simulink model "Lazurit_zarud_V2"  (R2018b)
settings: Solver=VariableStepAuto  StartTime=0.0  StopTime=2.5  RelTol=1e-3
undefined symbols (not defined in the file): Cout_filter_c, Cout_filter_r, Czpt_c, Czpt_r, delay_module_2, DiscIntNeverNeededParam, f, L_l, L_r, Lzpt_l, Lzpt_r, Rout, Ul, Uout, Uzpt
libraries: powerlib x60, powerlib_meascontrol x16, dspstat3 x11, simulink x4, simulink_extras x4, peRmsMeasurement x4
settings Model: Creator=VID Company  LastModifiedBy=VID Company

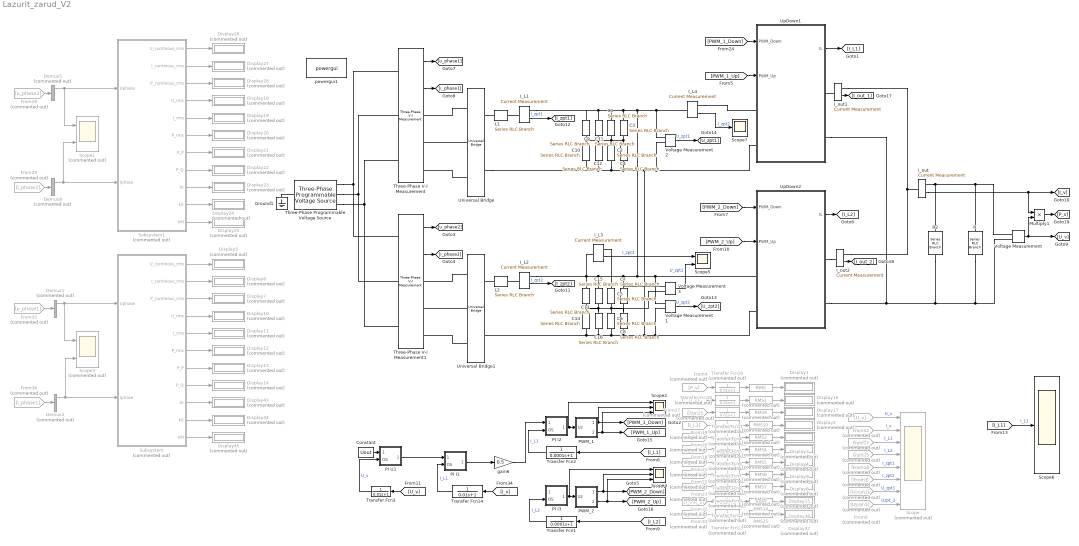
== system Lazurit_zarud_V2 ==
  C{1..16} (16 alike) : powerlib/Elements/Series RLC Branch  LConnTagsString=__new0  RConnTagsString=__new0  BranchType=RC  Resistance=Czpt_r  Inductance=1e-3  SetiL0=off  InitialCurrent=0  Capacitance=Czpt_c  Setx0=on  InitialVoltage=Uzpt/2  Measurements=Branch voltage
      settings: SourceProductName=Simscape Electrical
  Constant : Constant  Value=Uout
  Demux{1..2,5,8} (4 alike) : Demux  Commented=on  Outputs=3
  Display{1..28,37..38,43..45} (33 alike) : Display  Commented=on
  From1 : From  Commented=on  GotoTag=I_zpt1
  From12 : From  Commented=on  GotoTag=U_v
  From15 : From  Commented=on  GotoTag=I_L1
  From16 : From  Commented=on  GotoTag=I_L2
  From17 : From  Commented=on  GotoTag=I_v
  From18 : From  Commented=on  GotoTag=I_zpt1
  From19 : From  Commented=on  GotoTag=I_L1
  From2 : From  Commented=on  GotoTag=I_zpt2
  From20 : From  Commented=on  GotoTag=I_L2
  From21 : From  Commented=on  GotoTag=I_zpt2
  From22 : From  Commented=on  GotoTag=U_zpt1
  From23 : From  Commented=on  GotoTag=U_zpt2
  From25 : From  Commented=on  GotoTag=I_v
  From27 : From  Commented=on  GotoTag=U_v
  From28 : From  Commented=on  GotoTag=u_phase2
  From29 : From  Commented=on  GotoTag=i_phase2
  From3 : From  Commented=on  GotoTag=U_zpt1
  From32 : From  Commented=on  GotoTag=I_out_1
  From33 : From  Commented=on  GotoTag=I_out_2
  From35 : From  Commented=on  GotoTag=u_phase1
  From36 : From  Commented=on  GotoTag=i_phase1
  From4 : From  Commented=on  GotoTag=P_v
  From6 : From  Commented=on  GotoTag=U_zpt2
  Ground1 : powerlib/Elements/Ground  LConnTagsString=a
  I_L{1..4} (4 alike) : powerlib/Measurements/Current Measurement  PhasorSimulation=off  OutputType=Complex  PSBequivalent=0
      settings: SourceProductName=Simscape Electrical
  I_out : powerlib/Measurements/Current Measurement  PhasorSimulation=off  OutputType=Complex  PSBequivalent=0
      settings: SourceProductName=Simscape Electrical
  I_out1 : powerlib/Measurements/Current Measurement  PhasorSimulation=off  OutputType=Complex  PSBequivalent=0
      settings: SourceProductName=Simscape Electrical
  I_out2 : powerlib/Measurements/Current Measurement  PhasorSimulation=off  OutputType=Complex  PSBequivalent=0
      settings: SourceProductName=Simscape Electrical
  L1 : powerlib/Elements/Series RLC Branch  LConnTagsString=__new0  RConnTagsString=__new0  BranchType=RL  Resistance=Lzpt_r  Inductance=Lzpt_l  SetiL0=off  InitialCurrent=0  Capacitance=1e-6  Setx0=off  InitialVoltage=0  Measurements=None
      settings: SourceProductName=Simscape Electrical
  L2 : powerlib/Elements/Series RLC Branch  LConnTagsString=__new0  RConnTagsString=__new0  BranchType=RL  Resistance=Lzpt_r  Inductance=Lzpt_l  SetiL0=off  InitialCurrent=0  Capacitance=1e-6  Setx0=off  InitialVoltage=0  Measurements=None
      settings: SourceProductName=Simscape Electrical
  Multiply1 : Product
  PI I1 : Subsystem
  PI I2 : Subsystem
  PI I3 : Subsystem
  PI U1 : Subsystem
  PWM_1 : Subsystem
  PWM_2 : Subsystem
  R : powerlib/Elements/Series RLC Branch  LConnTagsString=__new0  RConnTagsString=__new0  BranchType=R  Resistance=Rout  Inductance=1e-3  SetiL0=off  InitialCurrent=0  Capacitance=6000e-6  Setx0=off  InitialVoltage=0  Measurements=None
  R2 : powerlib/Elements/Series RLC Branch  LConnTagsString=__new0  RConnTagsString=__new0  BranchType=R  Resistance=500  Inductance=1e-3  SetiL0=off  InitialCurrent=0  Capacitance=6000e-6  Setx0=off  InitialVoltage=0  Measurements=None
  RMS{1,3..10,14..15} (11 alike) : dspstat3/RMS  Commented=on  run=off  directionMode=Each column  dimension=1  InputProcessing=Columns as channels (frame based)  reset_popup=None
  Scope : Scope  Commented=on  NumInputPorts=8
  Scope1 : Scope  Commented=on  NumInputPorts=2
  Scope2 : Scope  NumInputPorts=3
  Scope3 : Scope  Commented=on  NumInputPorts=2
  Scope4 : Scope  NumInputPorts=3
  Scope5 : Scope  NumInputPorts=2
  Scope6 : Scope
  Scope7 : Scope
  Subsystem : Subsystem  Commented=on
  Subsystem1 : Subsystem  Commented=on
  Three-Phase Programmable Voltage Source : powerlib/Electrical Sources/Three-Phase Programmable Voltage Source  PositiveSequence=[Ul 0 50]  VariationEntity=None  VariationType=Table of time-amplitude pairs  VariationTypeAlt=Step  VariationStep=0.5  VariationRate=10  VariationMagnitude=0.3  VariationFrequency=2  VariationTiming=[1 2]  VariationPhaseA=off  Amplitudes=[1 0.8 1.2 1.0]  TimeValues=[0 0.1 0.15 0.2]  HarmonicGeneration=off  HarmonicA=[3 0.2 -25 0]  HarmonicB=[2 0.15 35 2]  Timing="[0.05  3]"  BusType=swing  Pref=0  Qref=0  Qmin=-inf  Qmax=inf
  Three-Phase V-I Measurement : powerlib/Measurements/Three-Phase V-I Measurement  VoltageMeasurement=phase-to-ground  SetLabelV=off  LabelV=Vabc  Vpu=off  VpuLL=off  CurrentMeasurement=yes  SetLabelI=off  LabelI=Iabc  Ipu=off  Pbase=100e6  Vbase=500e3  OutputType=Complex  PhasorSimulation=off  PSBequivalent=0
  Three-Phase V-I Measurement1 : powerlib/Measurements/Three-Phase V-I Measurement  VoltageMeasurement=phase-to-ground  SetLabelV=off  LabelV=Vabc  Vpu=off  VpuLL=off  CurrentMeasurement=yes  SetLabelI=off  LabelI=Iabc  Ipu=off  Pbase=100e6  Vbase=500e3  OutputType=Complex  PhasorSimulation=off  PSBequivalent=0
  Transfer Fcn1 : TransferFcn  Denominator=[0.0001 1]
  Transfer Fcn{4..13,19} (11 alike) : TransferFcn  Commented=on  Denominator=[0.01 1]
  Transfer Fcn14 : TransferFcn  Denominator=[0.01 1]
  Transfer Fcn2 : TransferFcn  Denominator=[0.0001 1]
  Transfer Fcn3 : TransferFcn  Denominator=[0.01 1]
  Universal Bridge : powerlib/Power Electronics/Universal Bridge  Arms=3  SnubberResistance=1e5  SnubberCapacitance=inf  Device=Diodes  Ron=Vd_r  Lon=0  ForwardVoltages="[  0  0  ]"  ForwardVoltage=Vd_v  GTOparameters=[ 10e-6 , 20e-6 ]  IGBTparameters=[ 1e-6 , 2e-6 ]  Measurements=None  Measurements_2=None  converterType=Rectifier
  Universal Bridge1 : powerlib/Power Electronics/Universal Bridge  Arms=3  SnubberResistance=1e5  SnubberCapacitance=inf  Device=Diodes  Ron=Vd_r  Lon=0  ForwardVoltages="[  0  0  ]"  ForwardVoltage=Vd_v  GTOparameters=[ 10e-6 , 20e-6 ]  IGBTparameters=[ 1e-6 , 2e-6 ]  Measurements=None  Measurements_2=None  converterType=Rectifier
  UpDown1 : Subsystem
  UpDown2 : Subsystem
  Voltage Measurement{,1..3} (4 alike) : powerlib/Measurements/Voltage Measurement  PhasorSimulation=off  OutputType=Complex  PSBequivalent=0
  gain6 : Gain  Gain=0.5  SaturateOnIntegerOverflow=on  OutDataTypeStr=Inherit: Same as input  ParamDataTypeStr=Inherit: Same as input
  powergui1 : powerlib/powergui  Priority=1  SimulationMode=Discrete  SampleTime=1e-6  frequency=60  Iterations=50  frequencyindice=50  Pbase=100e6  ErrMax=1e-4  UnitsV=kV  UnitsW=MW  buscounter=0  FunctionMessages=off  echomessages=off  EnableUseOfTLC=off  CurrentSourceSwitches=off  DisableSnubberDevices=off  DisableRonSwitches=off  DisableVfSwitches=off  DisplayEquations=off  SolverType=Tustin/Backward Euler (TBE)  Interpol=off  ExternalGateDelay=off  methode=off  Ts=100  x0status=blocks  SPID=on  SwTol=0  HookPort=off  RestoreLinks=warning  ResistiveCurrentMeasurement=off  Frange=[0:2:500]  Ylog=off  Xlog=on  ShowGrid=off  save=off  variable=ZData  structure=logsout  ZoomFFT=off  StartTime=0.1  cycles=30  DisplayStyle=2  fundamental=50  FreqAxis=off  MaxFrequency=1000  frequencyindicesteady=1  RmsSteady=1  display=off
  wires:
  Three-Phase V-I Measurement/1 -> [u_phase1]
  Three-Phase V-I Measurement1/1 -> [u_phase2]
  Three-Phase V-I Measurement/2 -> [i_phase1]
  Three-Phase V-I Measurement1/2 -> [i_phase2]
  PI I2/1(Out) -> Scope2/1, PWM_1/1(Uz)
  Transfer Fcn2/1 -> PI I2/2(OS)  "I_L1"
  Transfer Fcn1/1 -> PI I3/2(OS)  "I_L2"
  gain6/1 -> PI I2/1(Zad)
  PI I3/1(Out) -> Scope4/1, PWM_2/1(Uz)
  Constant/1 -> PI U1/1(Zad)
  Transfer Fcn3/1 -> PI U1/2(OS)  "U_v"
  PWM_1/1(CH1) -> Scope2/2, [PWM_1_Down]
  [I_L1] -> Transfer Fcn2/1
  PWM_2/1(CH1) -> Scope4/2, [PWM_2_Down]
  [I_L2] -> Transfer Fcn1/1
  Voltage Measurement/1 -> [U_v], Multiply1/2
  [U_v] -> Transfer Fcn3/1
  From12/1 -> Scope/1  "U_v"
  From15/1 -> Scope/3  "I_L1"
  From16/1 -> Scope/4  "I_L2"
  I_out/1 -> [I_v], Multiply1/1
  From17/1 -> Scope/2  "I_v"
  I_L2/1 -> [I_zpt2]  "I_zpt2"
  I_L1/1 -> [I_zpt1]  "I_zpt1"
  From1/1 -> Scope/5  "I_zpt1"
  From2/1 -> Scope/6  "I_zpt2"
  Voltage Measurement1/1 -> [U_zpt2]  "U_zpt2"
  From3/1 -> Scope/7  "U_zpt1"
  From6/1 -> Scope/8  "Uzpt_2"
  Multiply1/1 -> [P_v]
  From19/1 -> Transfer Fcn4/1
  From20/1 -> Transfer Fcn5/1
  From18/1 -> Transfer Fcn6/1
  From21/1 -> Transfer Fcn7/1
  From22/1 -> Transfer Fcn8/1
  From23/1 -> Transfer Fcn9/1
  RMS3/1 -> Display2/1
  RMS4/1 -> Display3/1
  RMS5/1 -> Display4/1
  RMS6/1 -> Display9/1
  RMS7/1 -> Display8/1
  RMS8/1 -> Display15/1
  Transfer Fcn4/1 -> RMS3/1
  Transfer Fcn5/1 -> RMS4/1
  Transfer Fcn6/1 -> RMS5/1
  Transfer Fcn7/1 -> RMS6/1
  Transfer Fcn8/1 -> RMS7/1
  Transfer Fcn9/1 -> RMS8/1
  PWM_1/2(CH2) -> Scope2/3, [PWM_1_Up]
  PWM_2/2(CH2) -> [PWM_2_Up], Scope4/3
  Transfer Fcn10/1 -> RMS9/1
  RMS9/1 -> Display16/1
  From25/1 -> Transfer Fcn10/1
  Transfer Fcn11/1 -> RMS10/1
  RMS10/1 -> Display17/1
  From27/1 -> Transfer Fcn11/1
  From33/1 -> Transfer Fcn13/1
  From32/1 -> Transfer Fcn12/1
  Transfer Fcn12/1 -> RMS14/1
  RMS14/1 -> Display38/1
  Transfer Fcn13/1 -> RMS15/1
  RMS15/1 -> Display37/1
  PI I1/1(Out) -> gain6/1
  PI U1/1(Out) -> PI I1/1(Zad)
  [I_v] -> Transfer Fcn14/1
  Transfer Fcn14/1 -> PI I1/2(OS)  "I_L1"
  Transfer Fcn19/1 -> RMS1/1
  RMS1/1 -> Display1/1
  From4/1 -> Transfer Fcn19/1
  Subsystem/1(U_continous_rms) -> Display5/1
  Subsystem/2(I_continous_rms) -> Display6/1
  Subsystem/3(P_continous_rms) -> Display7/1
  Subsystem/4(U_rms) -> Display10/1
  Subsystem/5(I_rms) -> Display11/1
  Subsystem/6(P_rms) -> Display12/1
  Subsystem/7(P_P) -> Display13/1
  Subsystem/8(P_Q) -> Display14/1
  Subsystem/9(kI) -> Display43/1
  Subsystem/10(kS) -> Display44/1
  Subsystem/11(kM) -> Display45/1
  Subsystem1/1(U_continous_rms) -> Display26/1
  Subsystem1/10(kS) -> Display24/1
  Subsystem1/3(P_continous_rms) -> Display28/1
  Subsystem1/7(P_P) -> Display21/1
  Subsystem1/6(P_rms) -> Display20/1
  Subsystem1/4(U_rms) -> Display18/1
  Subsystem1/2(I_continous_rms) -> Display27/1
  Subsystem1/9(kI) -> Display23/1
  Subsystem1/11(kM) -> Display25/1
  Subsystem1/5(I_rms) -> Display19/1
  Subsystem1/8(P_Q) -> Display22/1
  Voltage Measurement2/1 -> [U_zpt1]  "U_zpt1"
  [PWM_1_Down] -> UpDown1/1(PWM_Down)
  [PWM_1_Up] -> UpDown1/2(PWM_Up)
  [PWM_2_Down] -> UpDown2/1(PWM_Down)
  [PWM_2_Up] -> UpDown2/2(PWM_Up)
  UpDown1/1(IL) -> [I_L1]
  UpDown2/1(IL) -> [I_L2]
  I_out1/1 -> [I_out_1]
  I_out2/1 -> [I_out_2]
  Demux8/1 -> Subsystem1/2(Iphase), Scope1/2
  Demux5/1 -> Scope1/1, Subsystem1/1(Uphase)
  From28/1 -> Demux5/1
  From29/1 -> Demux8/1
  From35/1 -> Demux1/1
  From36/1 -> Demux2/1
  Demux1/1 -> Subsystem/1(Uphase), Scope3/1
  Demux2/1 -> Subsystem/2(Iphase), Scope3/2
  I_L3/1 -> Scope5/1  "I_zpt2"
  Voltage Measurement3/1 -> Scope5/2  "U_zpt2"
  [I_L1] -> Scope6/1  "I_L1"
  I_L4/1 -> Scope7/1  "I_zpt2"
  connections:
  Three-Phase Programmable Voltage Source/RConn3 -- Three-Phase V-I Measurement1/LConn3 -- Three-Phase V-I Measurement/LConn3
  Three-Phase Programmable Voltage Source/RConn1 -- Three-Phase V-I Measurement1/LConn1 -- Three-Phase V-I Measurement/LConn1
  Three-Phase Programmable Voltage Source/RConn2 -- Three-Phase V-I Measurement1/LConn2 -- Three-Phase V-I Measurement/LConn2
  Three-Phase Programmable Voltage Source/LConn1 -- Ground1/LConn1
  Universal Bridge/LConn1 -- Three-Phase V-I Measurement/RConn1
  Universal Bridge/LConn2 -- Three-Phase V-I Measurement/RConn2
  Universal Bridge/LConn3 -- Three-Phase V-I Measurement/RConn3
  I_out/RConn1 -- R2/LConn1 -- R/LConn1 -- Voltage Measurement/LConn1
  L1/LConn1 -- Universal Bridge/RConn1
  L2/LConn1 -- Universal Bridge1/RConn1
  Universal Bridge1/LConn1 -- Three-Phase V-I Measurement1/RConn1
  Universal Bridge1/LConn2 -- Three-Phase V-I Measurement1/RConn2
  Universal Bridge1/LConn3 -- Three-Phase V-I Measurement1/RConn3
  I_L2/RConn1 -- C15/LConn1 -- Voltage Measurement3/LConn1 -- C7/LConn1 -- I_L4/LConn1 -- Voltage Measurement2/LConn1 -- C9/LConn1 -- I_L1/RConn1 -- C11/LConn1 -- C1/LConn1 -- C3/LConn1 -- UpDown2/LConn1 -- Voltage Measurement1/LConn1 -- I_L3/LConn1 -- C13/LConn1
  I_L2/LConn1 -- L2/RConn1
  I_L1/LConn1 -- L1/RConn1
  UpDown2/RConn2 -- UpDown1/RConn2 -- R2/RConn1 -- R/RConn1 -- Voltage Measurement/LConn2
  C13/RConn1 -- C16/LConn1 -- C6/LConn1 -- C8/LConn1 -- Voltage Measurement3/LConn2 -- C7/RConn1 -- C5/RConn1 -- C15/RConn1 -- C14/LConn1
  I_out1/LConn1 -- UpDown1/RConn1
  I_out1/RConn1 -- I_out2/RConn1 -- I_out/LConn1
  UpDown2/RConn1 -- I_out2/LConn1
  I_L3/RConn1 -- C5/LConn1
  C3/RConn1 -- C11/RConn1 -- C12/LConn1 -- C10/LConn1 -- C9/RConn1 -- C2/LConn1 -- C1/RConn1 -- C4/LConn1
  UpDown2/LConn2 -- Voltage Measurement1/LConn2 -- UpDown1/LConn2 -- Voltage Measurement2/LConn2 -- C4/RConn1 -- C12/RConn1 -- C10/RConn1 -- Universal Bridge/RConn2 -- C2/RConn1 -- C8/RConn1 -- C6/RConn1 -- C16/RConn1 -- C14/RConn1 -- Universal Bridge1/RConn2
  I_L4/RConn1 -- UpDown1/LConn1

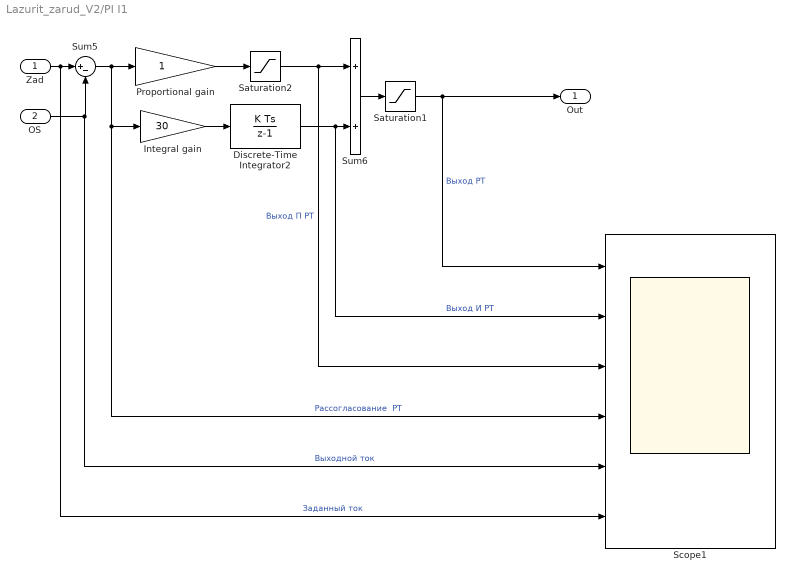
== system Lazurit_zarud_V2/PI I1 ==
  Zad : Inport
  OS : Inport  Port=2
  Discrete-Time Integrator2 : DiscreteIntegrator  SampleTime=-1  LimitOutput=on  UpperSaturationLimit=260  LowerSaturationLimit=0  ICPrevOutput=DiscIntNeverNeededParam  ICPrevScaledInput=DiscIntNeverNeededParam
  Integral gain : Gain  Gain=30  SaturateOnIntegerOverflow=on  OutDataTypeStr=Inherit: Same as input  ParamDataTypeStr=Inherit: Same as input
  Proportional gain : Gain  SaturateOnIntegerOverflow=on  OutDataTypeStr=Inherit: Same as input  ParamDataTypeStr=Inherit: Same as input
  Saturation1 : Saturate  UpperLimit=260  LowerLimit=0
  Saturation2 : Saturate  UpperLimit=250  LowerLimit=-250
  Scope1 : Scope  NumInputPorts=6
  Sum5 : Sum  Inputs=|+-  SaturateOnIntegerOverflow=on  InputSameDT=on  OutDataTypeStr=Inherit: Same as first input
  Sum6 : Sum  SaturateOnIntegerOverflow=on  InputSameDT=on  OutDataTypeStr=Inherit: Same as first input
  Out : Outport
  wires:
  Integral gain/1 -> Discrete-Time Integrator2/1
  Discrete-Time Integrator2/1 -> Scope1/2, Sum6/2  "Выход И РТ"
  OS/1 -> Scope1/5, Sum5/2  "Выходной ток"
  Zad/1 -> Scope1/6, Sum5/1  "Заданный ток"
  Sum5/1 -> Scope1/4, Integral gain/1, Proportional gain/1  "Рассогласование  РТ"
  Sum6/1 -> Saturation1/1
  Saturation1/1 -> Out/1, Scope1/1  "Выход РТ"
  Proportional gain/1 -> Saturation2/1
  Saturation2/1 -> Scope1/3, Sum6/1  "Выход П РТ"

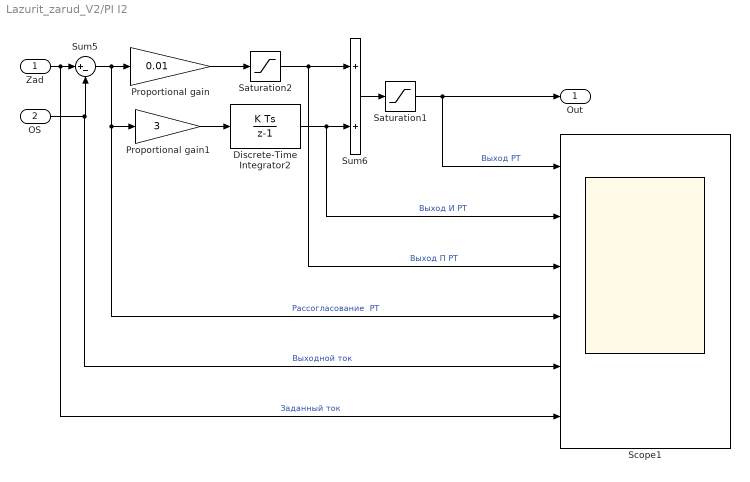
== system Lazurit_zarud_V2/PI I2 ==
  Zad : Inport
  OS : Inport  Port=2
  Discrete-Time Integrator2 : DiscreteIntegrator  SampleTime=-1  LimitOutput=on  UpperSaturationLimit=1.35  LowerSaturationLimit=0  ICPrevOutput=DiscIntNeverNeededParam  ICPrevScaledInput=DiscIntNeverNeededParam
  Proportional gain : Gain  Gain=0.01  SaturateOnIntegerOverflow=on  OutDataTypeStr=Inherit: Same as input  ParamDataTypeStr=Inherit: Same as input
  Proportional gain1 : Gain  Gain=3  SaturateOnIntegerOverflow=on  OutDataTypeStr=Inherit: Same as input  ParamDataTypeStr=Inherit: Same as input
  Saturation1 : Saturate  UpperLimit=1.2  LowerLimit=0
  Saturation2 : Saturate  UpperLimit=0.3  LowerLimit=-0.8
  Scope1 : Scope  NumInputPorts=6
  Sum5 : Sum  Inputs=|+-  SaturateOnIntegerOverflow=on  InputSameDT=on  OutDataTypeStr=Inherit: Same as first input
  Sum6 : Sum  SaturateOnIntegerOverflow=on  InputSameDT=on  OutDataTypeStr=Inherit: Same as first input
  Out : Outport
  wires:
  Proportional gain/1 -> Saturation2/1
  Discrete-Time Integrator2/1 -> Sum6/2, Scope1/2  "Выход И РТ"
  OS/1 -> Scope1/5, Sum5/2  "Выходной ток"
  Zad/1 -> Scope1/6, Sum5/1  "Заданный ток"
  Sum5/1 -> Proportional gain1/1, Scope1/4, Proportional gain/1  "Рассогласование  РТ"
  Sum6/1 -> Saturation1/1
  Saturation1/1 -> Out/1, Scope1/1  "Выход РТ"
  Proportional gain1/1 -> Discrete-Time Integrator2/1
  Saturation2/1 -> Scope1/3, Sum6/1  "Выход П РТ"

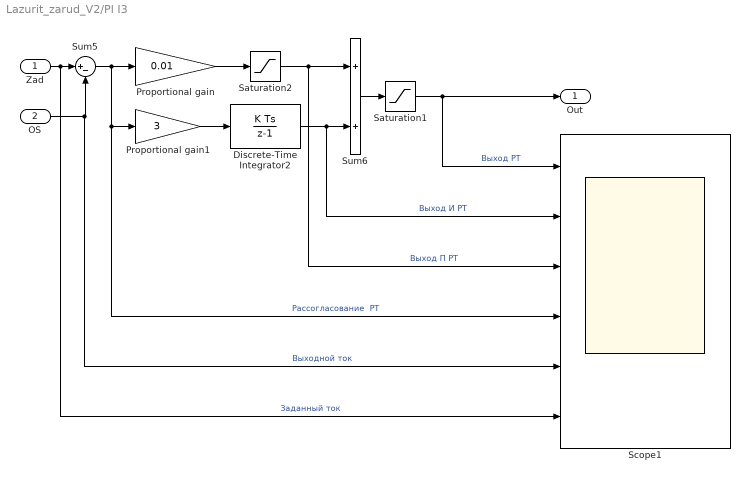
== system Lazurit_zarud_V2/PI I3 ==
  Zad : Inport
  OS : Inport  Port=2
  Discrete-Time Integrator2 : DiscreteIntegrator  SampleTime=-1  LimitOutput=on  UpperSaturationLimit=1.35  LowerSaturationLimit=0  ICPrevOutput=DiscIntNeverNeededParam  ICPrevScaledInput=DiscIntNeverNeededParam
  Proportional gain : Gain  Gain=0.01  SaturateOnIntegerOverflow=on  OutDataTypeStr=Inherit: Same as input  ParamDataTypeStr=Inherit: Same as input
  Proportional gain1 : Gain  Gain=3  SaturateOnIntegerOverflow=on  OutDataTypeStr=Inherit: Same as input  ParamDataTypeStr=Inherit: Same as input
  Saturation1 : Saturate  UpperLimit=1.35  LowerLimit=0
  Saturation2 : Saturate  UpperLimit=0.3  LowerLimit=-0.8
  Scope1 : Scope  NumInputPorts=6
  Sum5 : Sum  Inputs=|+-  SaturateOnIntegerOverflow=on  InputSameDT=on  OutDataTypeStr=Inherit: Same as first input
  Sum6 : Sum  SaturateOnIntegerOverflow=on  InputSameDT=on  OutDataTypeStr=Inherit: Same as first input
  Out : Outport
  wires:
  Proportional gain/1 -> Saturation2/1
  Discrete-Time Integrator2/1 -> Sum6/2, Scope1/2  "Выход И РТ"
  OS/1 -> Scope1/5, Sum5/2  "Выходной ток"
  Zad/1 -> Scope1/6, Sum5/1  "Заданный ток"
  Sum5/1 -> Proportional gain1/1, Scope1/4, Proportional gain/1  "Рассогласование  РТ"
  Sum6/1 -> Saturation1/1
  Saturation1/1 -> Out/1, Scope1/1  "Выход РТ"
  Proportional gain1/1 -> Discrete-Time Integrator2/1
  Saturation2/1 -> Scope1/3, Sum6/1  "Выход П РТ"

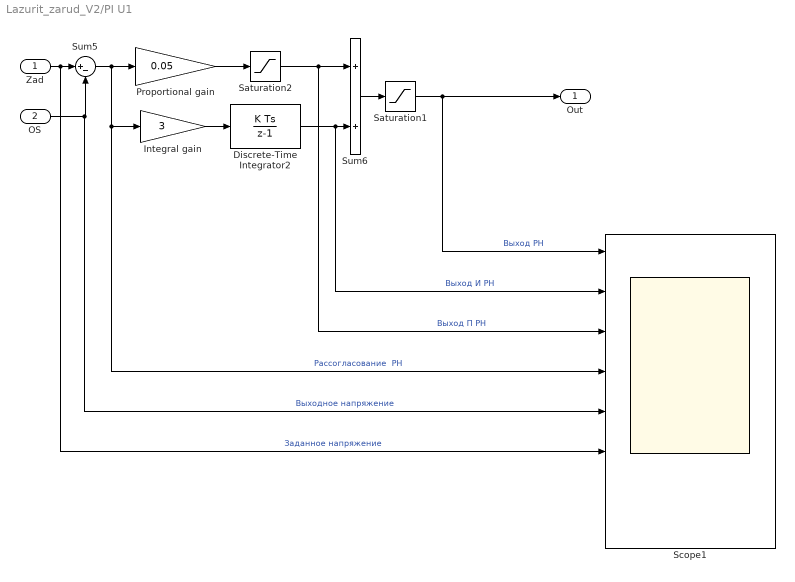
== system Lazurit_zarud_V2/PI U1 ==
  Zad : Inport
  OS : Inport  Port=2
  Discrete-Time Integrator2 : DiscreteIntegrator  SampleTime=-1  LimitOutput=on  UpperSaturationLimit=250  LowerSaturationLimit=0  ICPrevOutput=DiscIntNeverNeededParam  ICPrevScaledInput=DiscIntNeverNeededParam
  Integral gain : Gain  Gain=3  SaturateOnIntegerOverflow=on  OutDataTypeStr=Inherit: Same as input  ParamDataTypeStr=Inherit: Same as input
  Proportional gain : Gain  Gain=0.05  SaturateOnIntegerOverflow=on  OutDataTypeStr=Inherit: Same as input  ParamDataTypeStr=Inherit: Same as input
  Saturation1 : Saturate  UpperLimit=250  LowerLimit=0
  Saturation2 : Saturate  UpperLimit=250  LowerLimit=-250
  Scope1 : Scope  NumInputPorts=8
  Sum5 : Sum  Inputs=|+-  SaturateOnIntegerOverflow=on  InputSameDT=on  OutDataTypeStr=Inherit: Same as first input
  Sum6 : Sum  SaturateOnIntegerOverflow=on  InputSameDT=on  OutDataTypeStr=Inherit: Same as first input
  Out : Outport
  wires:
  Integral gain/1 -> Discrete-Time Integrator2/1
  Discrete-Time Integrator2/1 -> Scope1/2, Sum6/2  "Выход И РН"
  OS/1 -> Scope1/5, Sum5/2  "Выходное напряжение"
  Zad/1 -> Scope1/6, Sum5/1  "Заданное напряжение"
  Sum5/1 -> Scope1/4, Integral gain/1, Proportional gain/1  "Рассогласование  РН"
  Sum6/1 -> Saturation1/1
  Saturation1/1 -> Out/1, Scope1/1  "Выход РН"
  Proportional gain/1 -> Saturation2/1
  Saturation2/1 -> Scope1/3, Sum6/1  "Выход П РН"

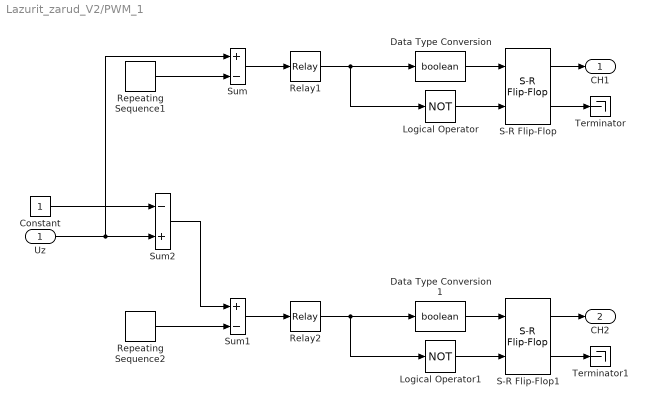
== system Lazurit_zarud_V2/PWM_1 ==
  Uz : Inport
  Constant : Constant
  Data Type Conversion : DataTypeConversion  OutDataTypeStr=boolean
  Data Type Conversion1 : DataTypeConversion  OutDataTypeStr=boolean
  Logical Operator : Logic  Operator=NOT  AllPortsSameDT=off  OutDataTypeStr=boolean
  Logical Operator1 : Logic  Operator=NOT  AllPortsSameDT=off  OutDataTypeStr=boolean
  Relay1 : Relay  OnSwitchValue=0.01  OffSwitchValue=-0.01
  Relay2 : Relay  OnSwitchValue=0.01  OffSwitchValue=-0.01
  Repeating Sequence1 : simulink/Sources/Repeating Sequence  rep_seq_t="[0  (1/(2*f)) (1/f)]"  rep_seq_y=[0 1 0]
  Repeating Sequence2 : simulink/Sources/Repeating Sequence  rep_seq_t="[0  (1/(2*f)) (1/f)]"  rep_seq_y=[0 1 0]
  S-R Flip-Flop : simulink_extras/Flip Flops/S-R Flip-Flop  initial_condition=0
  S-R Flip-Flop1 : simulink_extras/Flip Flops/S-R Flip-Flop  initial_condition=0
  Sum : Sum  Inputs=+-
  Sum1 : Sum  Inputs=+-
  Sum2 : Sum  Inputs=-+
  Terminator : Terminator
  Terminator1 : Terminator
  CH1 : Outport
  CH2 : Outport  Port=2
  wires:
  S-R Flip-Flop/1 -> CH1/1
  Data Type Conversion/1 -> S-R Flip-Flop/1
  Logical Operator/1 -> S-R Flip-Flop/2
  Relay1/1 -> Logical Operator/1, Data Type Conversion/1
  Repeating Sequence1/1 -> Sum/2
  Sum/1 -> Relay1/1
  S-R Flip-Flop/2 -> Terminator/1
  Data Type Conversion1/1 -> S-R Flip-Flop1/1
  Logical Operator1/1 -> S-R Flip-Flop1/2
  S-R Flip-Flop1/2 -> Terminator1/1
  Relay2/1 -> Logical Operator1/1, Data Type Conversion1/1
  S-R Flip-Flop1/1 -> CH2/1
  Sum1/1 -> Relay2/1
  Uz/1 -> Sum/1, Sum2/2
  Constant/1 -> Sum2/1
  Sum2/1 -> Sum1/1
  Repeating Sequence2/1 -> Sum1/2

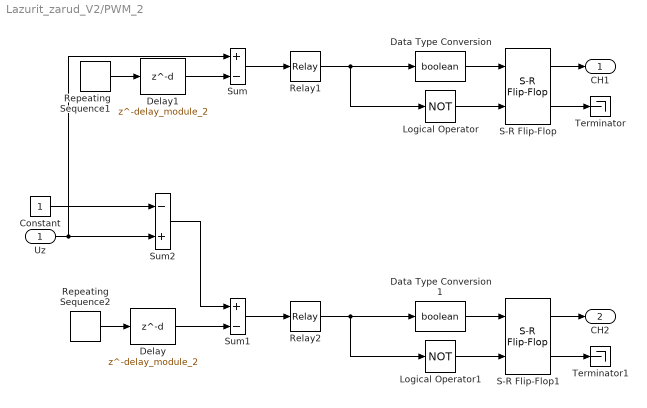
== system Lazurit_zarud_V2/PWM_2 ==
  Uz : Inport
  Constant : Constant
  Data Type Conversion : DataTypeConversion  OutDataTypeStr=boolean
  Data Type Conversion1 : DataTypeConversion  OutDataTypeStr=boolean
  Delay : Delay  DelayLength=delay_module_2
  Delay1 : Delay  DelayLength=delay_module_2
  Logical Operator : Logic  Operator=NOT  AllPortsSameDT=off  OutDataTypeStr=boolean
  Logical Operator1 : Logic  Operator=NOT  AllPortsSameDT=off  OutDataTypeStr=boolean
  Relay1 : Relay  OnSwitchValue=0.01  OffSwitchValue=-0.01
  Relay2 : Relay  OnSwitchValue=0.01  OffSwitchValue=-0.01
  Repeating Sequence1 : simulink/Sources/Repeating Sequence  rep_seq_t="[0  (1/(2*f)) (1/f)]"  rep_seq_y=[0 1 0]
  Repeating Sequence2 : simulink/Sources/Repeating Sequence  rep_seq_t="[0  (1/(2*f)) (1/f)]"  rep_seq_y=[0 1 0]
  S-R Flip-Flop : simulink_extras/Flip Flops/S-R Flip-Flop  initial_condition=0
  S-R Flip-Flop1 : simulink_extras/Flip Flops/S-R Flip-Flop  initial_condition=0
  Sum : Sum  Inputs=+-
  Sum1 : Sum  Inputs=+-
  Sum2 : Sum  Inputs=-+
  Terminator : Terminator
  Terminator1 : Terminator
  CH1 : Outport
  CH2 : Outport  Port=2
  wires:
  S-R Flip-Flop/1 -> CH1/1
  Data Type Conversion/1 -> S-R Flip-Flop/1
  Logical Operator/1 -> S-R Flip-Flop/2
  Relay1/1 -> Logical Operator/1, Data Type Conversion/1
  Sum/1 -> Relay1/1
  S-R Flip-Flop/2 -> Terminator/1
  Data Type Conversion1/1 -> S-R Flip-Flop1/1
  Logical Operator1/1 -> S-R Flip-Flop1/2
  S-R Flip-Flop1/2 -> Terminator1/1
  Relay2/1 -> Logical Operator1/1, Data Type Conversion1/1
  S-R Flip-Flop1/1 -> CH2/1
  Sum1/1 -> Relay2/1
  Repeating Sequence2/1 -> Delay/1
  Uz/1 -> Sum2/2, Sum/1
  Constant/1 -> Sum2/1
  Sum2/1 -> Sum1/1
  Delay/1 -> Sum1/2
  Repeating Sequence1/1 -> Delay1/1
  Delay1/1 -> Sum/2

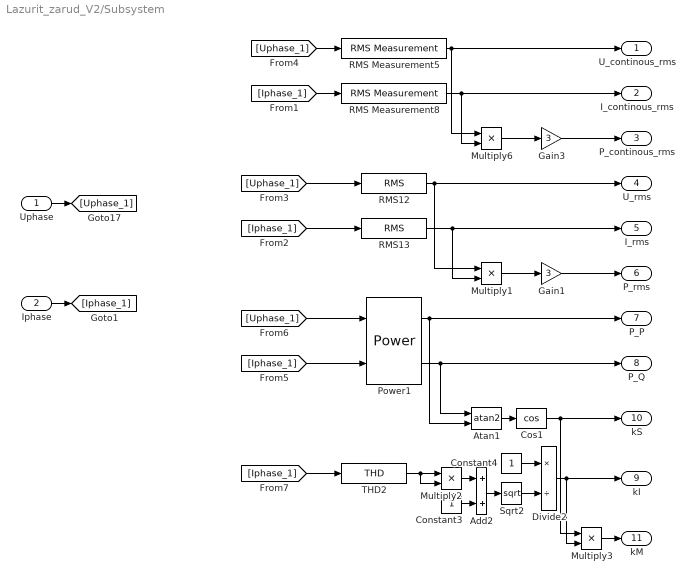
== system Lazurit_zarud_V2/Subsystem ==
  Uphase : Inport
  Iphase : Inport  Port=2
  Add2 : Sum
  Atan1 : Trigonometry  Operator=atan2
  Constant3 : Constant
  Constant4 : Constant
  Cos1 : Trigonometry  Operator=cos
  Divide2 : Product  Inputs=*/
  Gain1 : Gain  Gain=3
  Gain3 : Gain  Gain=3
  Multiply{1..3,6} (4 alike) : Product
  Power1 : powerlib_meascontrol/Measurements/Power  Freq=50  Vinit=[1, 0]  Iinit=[1, 0]  Ts=0
      settings: SourceProductName=Simscape Power Systems
  RMS Measurement5 : peRmsMeasurement/RMS Measurement  LabelModeActiveChoice=Harmonic  F=50  SpecifyHarmonics=on  K=[1]  Ts=0
  RMS Measurement8 : peRmsMeasurement/RMS Measurement  LabelModeActiveChoice=Harmonic  F=50  SpecifyHarmonics=on  K=[1]  Ts=0
  RMS12 : powerlib_meascontrol/Measurements/RMS  TrueRMS=on  Freq=50  RMSInit=0  Ts=0
  RMS13 : powerlib_meascontrol/Measurements/RMS  TrueRMS=on  Freq=50  RMSInit=0  Ts=0
  Sqrt2 : Sqrt  SaturateOnIntegerOverflow=on
  THD2 : powerlib_meascontrol/Measurements/THD  Freq=50  Ts=0
  U_continous_rms : Outport
  I_continous_rms : Outport  Port=2
  P_continous_rms : Outport  Port=3
  U_rms : Outport  Port=4
  I_rms : Outport  Port=5
  P_rms : Outport  Port=6
  P_P : Outport  Port=7
  P_Q : Outport  Port=8
  kI : Outport  Port=9
  kS : Outport  Port=10
  kM : Outport  Port=11
  wires:
  RMS Measurement5/1 -> Multiply6/1, U_continous_rms/1
  RMS Measurement8/1 -> Multiply6/2, I_continous_rms/1
  [Uphase_1] -> RMS Measurement5/1
  [Iphase_1] -> RMS Measurement8/1
  Multiply6/1 -> Gain3/1
  RMS12/1 -> Multiply1/1, U_rms/1
  [Uphase_1] -> RMS12/1
  [Iphase_1] -> RMS13/1
  RMS13/1 -> Multiply1/2, I_rms/1
  Multiply1/1 -> Gain1/1
  Atan1/1 -> Cos1/1
  Power1/1 -> Atan1/2, P_P/1
  Power1/2 -> Atan1/1, P_Q/1
  [Uphase_1] -> Power1/1
  [Iphase_1] -> Power1/2
  Cos1/1 -> Multiply3/1, kS/1
  Sqrt2/1 -> Divide2/2
  THD2/1 -> Multiply2/1, Multiply2/2
  Constant3/1 -> Add2/2
  Multiply2/1 -> Add2/1
  Constant4/1 -> Divide2/1
  Divide2/1 -> Multiply3/2, kI/1
  Add2/1 -> Sqrt2/1
  [Iphase_1] -> THD2/1
  Multiply3/1 -> kM/1
  Gain3/1 -> P_continous_rms/1
  Gain1/1 -> P_rms/1
  Uphase/1 -> [Uphase_1]
  Iphase/1 -> [Iphase_1]

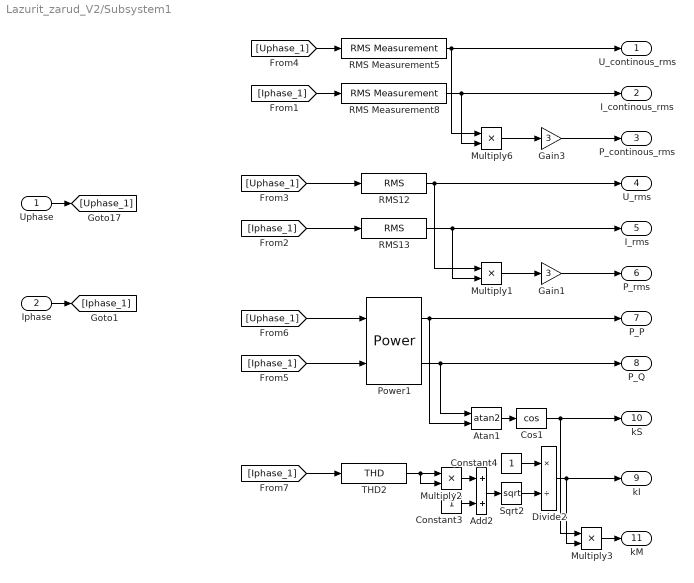
== system Lazurit_zarud_V2/Subsystem1 ==
  Uphase : Inport
  Iphase : Inport  Port=2
  Add2 : Sum
  Atan1 : Trigonometry  Operator=atan2
  Constant3 : Constant
  Constant4 : Constant
  Cos1 : Trigonometry  Operator=cos
  Divide2 : Product  Inputs=*/
  Gain1 : Gain  Gain=3
  Gain3 : Gain  Gain=3
  Multiply{1..3,6} (4 alike) : Product
  Power1 : powerlib_meascontrol/Measurements/Power  Freq=50  Vinit=[1, 0]  Iinit=[1, 0]  Ts=0
      settings: SourceProductName=Simscape Power Systems
  RMS Measurement5 : peRmsMeasurement/RMS Measurement  LabelModeActiveChoice=Harmonic  F=50  SpecifyHarmonics=on  K=[1]  Ts=0
  RMS Measurement8 : peRmsMeasurement/RMS Measurement  LabelModeActiveChoice=Harmonic  F=50  SpecifyHarmonics=on  K=[1]  Ts=0
  RMS12 : powerlib_meascontrol/Measurements/RMS  TrueRMS=on  Freq=50  RMSInit=0  Ts=0
  RMS13 : powerlib_meascontrol/Measurements/RMS  TrueRMS=on  Freq=50  RMSInit=0  Ts=0
  Sqrt2 : Sqrt  SaturateOnIntegerOverflow=on
  THD2 : powerlib_meascontrol/Measurements/THD  Freq=50  Ts=0
  U_continous_rms : Outport
  I_continous_rms : Outport  Port=2
  P_continous_rms : Outport  Port=3
  U_rms : Outport  Port=4
  I_rms : Outport  Port=5
  P_rms : Outport  Port=6
  P_P : Outport  Port=7
  P_Q : Outport  Port=8
  kI : Outport  Port=9
  kS : Outport  Port=10
  kM : Outport  Port=11
  wires:
  RMS Measurement5/1 -> Multiply6/1, U_continous_rms/1
  RMS Measurement8/1 -> Multiply6/2, I_continous_rms/1
  [Uphase_1] -> RMS Measurement5/1
  [Iphase_1] -> RMS Measurement8/1
  Multiply6/1 -> Gain3/1
  RMS12/1 -> Multiply1/1, U_rms/1
  [Uphase_1] -> RMS12/1
  [Iphase_1] -> RMS13/1
  RMS13/1 -> Multiply1/2, I_rms/1
  Multiply1/1 -> Gain1/1
  Atan1/1 -> Cos1/1
  Power1/1 -> Atan1/2, P_P/1
  Power1/2 -> Atan1/1, P_Q/1
  [Uphase_1] -> Power1/1
  [Iphase_1] -> Power1/2
  Cos1/1 -> Multiply3/1, kS/1
  Sqrt2/1 -> Divide2/2
  THD2/1 -> Multiply2/1, Multiply2/2
  Constant3/1 -> Add2/2
  Multiply2/1 -> Add2/1
  Constant4/1 -> Divide2/1
  Divide2/1 -> Multiply3/2, kI/1
  Add2/1 -> Sqrt2/1
  [Iphase_1] -> THD2/1
  Multiply3/1 -> kM/1
  Gain3/1 -> P_continous_rms/1
  Gain1/1 -> P_rms/1
  Uphase/1 -> [Uphase_1]
  Iphase/1 -> [Iphase_1]

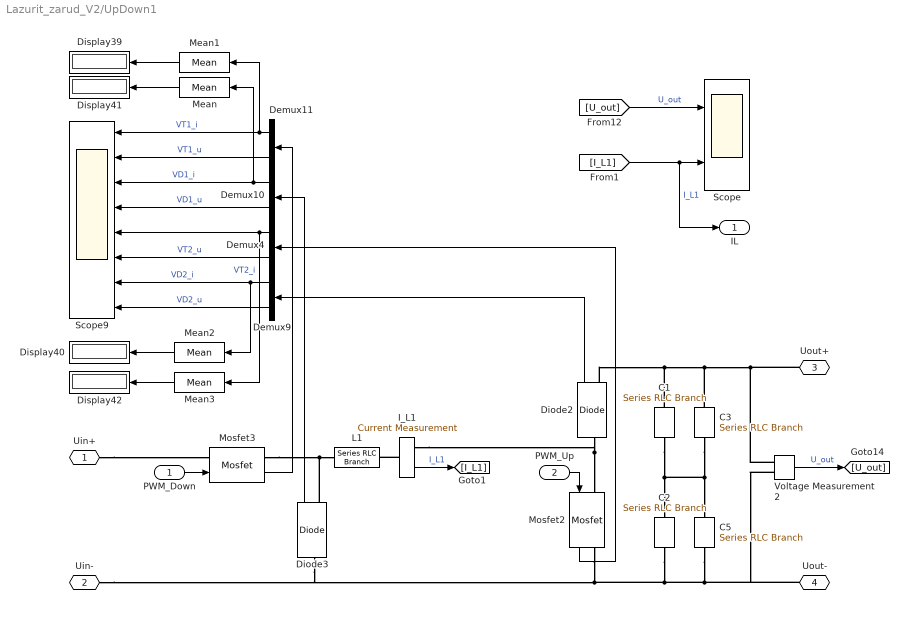
== system Lazurit_zarud_V2/UpDown1 ==
  PWM_Down : Inport
  PWM_Up : Inport  Port=2
  C{1..3,5} (4 alike) : powerlib/Elements/Series RLC Branch  LConnTagsString=__new0  RConnTagsString=__new0  BranchType=RC  Resistance=Cout_filter_r  Inductance=1e-3  SetiL0=off  InitialCurrent=0  Capacitance=Cout_filter_c  Setx0=on  InitialVoltage=0  Measurements=Branch voltage
      settings: SourceProductName=Simscape Electrical
  Demux{4,9..11} (4 alike) : Demux  Outputs=2
  Diode2 : powerlib/Power Electronics/Diode  Ron=0.001  Lon=0  Vf=0.8  IC=0  UseSnubber=off  Rs=500  Cs=250e-9  Measurements=on
      settings: SourceProductName=Simscape Electrical
  Diode3 : powerlib/Power Electronics/Diode  Ron=0.001  Lon=0  Vf=0.8  IC=0  UseSnubber=off  Rs=500  Cs=250e-9  Measurements=on
      settings: SourceProductName=Simscape Electrical
  Display{39..42} (4 alike) : Display
  I_L1 : powerlib/Measurements/Current Measurement  PhasorSimulation=off  OutputType=Complex  PSBequivalent=0
      settings: SourceProductName=Simscape Electrical
  L1 : powerlib/Elements/Series RLC Branch  LConnTagsString=__new0  RConnTagsString=__new0  BranchType=RL  Resistance=L_r  Inductance=L_l  SetiL0=off  InitialCurrent=0  Capacitance=1e-6  Setx0=off  InitialVoltage=0  Measurements=None
      settings: SourceProductName=Simscape Electrical
  Mean{,1..3} (4 alike) : powerlib_meascontrol/Measurements/Mean  Freq=f  Vinit=0  Ts=0
  Mosfet2 : powerlib/Power Electronics/Mosfet  Ron=1e-6  Lon=0  Rd=1e-6  Vfd=0  IC=0  Rs=1e5  Cs=inf  Measurements=on
      settings: SourceProductName=Simscape Electrical
  Mosfet3 : powerlib/Power Electronics/Mosfet  Ron=1e-6  Lon=0  Rd=1e-6  Vfd=0  IC=0  Rs=1e5  Cs=inf  Measurements=on
      settings: SourceProductName=Simscape Electrical
  Scope : Scope  NumInputPorts=2
  Scope9 : Scope  NumInputPorts=8
  Voltage Measurement2 : powerlib/Measurements/Voltage Measurement  PhasorSimulation=off  OutputType=Complex  PSBequivalent=0
  Uin+ : PMIOPort  Side=Left
  Uin- : PMIOPort  Port=2  Side=Left
  Uout+ : PMIOPort  Port=3  Side=Right
  Uout- : PMIOPort  Port=4  Side=Right
  IL : Outport
  wires:
  Demux4/1 -> Mean3/1, Scope9/5  "VT2_i"
  Demux9/1 -> Mean2/1, Scope9/7  "VD2_i"
  Demux11/2 -> Scope9/2  "VT1_u"
  PWM_Down/1 -> Mosfet3/1
  Demux10/1 -> Mean/1, Scope9/3  "VD1_i"
  Demux11/1 -> Mean1/1, Scope9/1  "VT1_i"
  Demux10/2 -> Scope9/4  "VD1_u"
  Diode3/1 -> Demux10/1
  Demux9/2 -> Scope9/8  "VD2_u"
  PWM_Up/1 -> Mosfet2/1
  Mosfet2/1 -> Demux4/1
  Demux4/2 -> Scope9/6  "VT2_u"
  Mosfet3/1 -> Demux11/1
  Diode2/1 -> Demux9/1
  I_L1/1 -> [I_L1]  "I_L1"
  Mean1/1 -> Display39/1
  Mean/1 -> Display41/1
  Mean2/1 -> Display40/1
  Mean3/1 -> Display42/1
  Voltage Measurement2/1 -> [U_out]  "U_out"
  [U_out] -> Scope/1  "U_out"
  [I_L1] -> IL/1, Scope/2  "I_L1"
  connections:
  Uin+/RConn1 -- Mosfet3/LConn1
  Diode2/RConn1 -- C1/LConn1 -- C3/LConn1 -- Voltage Measurement2/LConn1 -- Uout+/RConn1
  I_L1/RConn1 -- Diode2/LConn1 -- Mosfet2/LConn1
  Diode3/RConn1 -- L1/LConn1 -- Mosfet3/RConn1
  Mosfet2/RConn1 -- C5/RConn1 -- Voltage Measurement2/LConn2 -- Uout-/RConn1 -- C2/RConn1 -- Uin-/RConn1 -- Diode3/LConn1
  I_L1/LConn1 -- L1/RConn1
  C3/RConn1 -- C2/LConn1 -- C1/RConn1 -- C5/LConn1

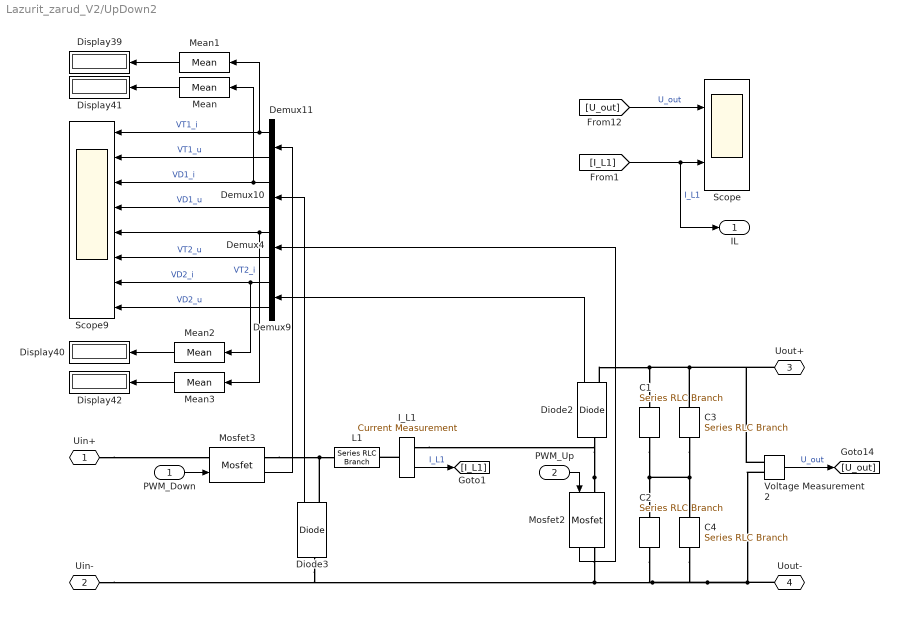
== system Lazurit_zarud_V2/UpDown2 ==
  PWM_Down : Inport
  PWM_Up : Inport  Port=2
  C{1..4} (4 alike) : powerlib/Elements/Series RLC Branch  LConnTagsString=__new0  RConnTagsString=__new0  BranchType=RC  Resistance=Cout_filter_r  Inductance=1e-3  SetiL0=off  InitialCurrent=0  Capacitance=Cout_filter_c  Setx0=on  InitialVoltage=0  Measurements=Branch voltage
      settings: SourceProductName=Simscape Electrical
  Demux{4,9..11} (4 alike) : Demux  Outputs=2
  Diode2 : powerlib/Power Electronics/Diode  Ron=0.001  Lon=0  Vf=0.8  IC=0  UseSnubber=off  Rs=500  Cs=250e-9  Measurements=on
      settings: SourceProductName=Simscape Electrical
  Diode3 : powerlib/Power Electronics/Diode  Ron=0.001  Lon=0  Vf=0.8  IC=0  UseSnubber=off  Rs=500  Cs=250e-9  Measurements=on
      settings: SourceProductName=Simscape Electrical
  Display{39..42} (4 alike) : Display
  I_L1 : powerlib/Measurements/Current Measurement  PhasorSimulation=off  OutputType=Complex  PSBequivalent=0
      settings: SourceProductName=Simscape Electrical
  L1 : powerlib/Elements/Series RLC Branch  LConnTagsString=__new0  RConnTagsString=__new0  BranchType=RL  Resistance=L_r  Inductance=L_l  SetiL0=off  InitialCurrent=0  Capacitance=1e-6  Setx0=off  InitialVoltage=0  Measurements=None
      settings: SourceProductName=Simscape Electrical
  Mean{,1..3} (4 alike) : powerlib_meascontrol/Measurements/Mean  Freq=f  Vinit=0  Ts=0
  Mosfet2 : powerlib/Power Electronics/Mosfet  Ron=1e-6  Lon=0  Rd=1e-6  Vfd=0  IC=0  Rs=1e5  Cs=inf  Measurements=on
      settings: SourceProductName=Simscape Electrical
  Mosfet3 : powerlib/Power Electronics/Mosfet  Ron=1e-6  Lon=0  Rd=1e-6  Vfd=0  IC=0  Rs=1e5  Cs=inf  Measurements=on
      settings: SourceProductName=Simscape Electrical
  Scope : Scope  NumInputPorts=2
  Scope9 : Scope  NumInputPorts=8
  Voltage Measurement2 : powerlib/Measurements/Voltage Measurement  PhasorSimulation=off  OutputType=Complex  PSBequivalent=0
  Uin+ : PMIOPort  Side=Left
  Uin- : PMIOPort  Port=2  Side=Left
  Uout+ : PMIOPort  Port=3  Side=Right
  Uout- : PMIOPort  Port=4  Side=Right
  IL : Outport
  wires:
  Demux4/1 -> Mean3/1, Scope9/5  "VT2_i"
  Demux9/1 -> Mean2/1, Scope9/7  "VD2_i"
  Demux11/2 -> Scope9/2  "VT1_u"
  PWM_Down/1 -> Mosfet3/1
  Demux10/1 -> Mean/1, Scope9/3  "VD1_i"
  Demux11/1 -> Mean1/1, Scope9/1  "VT1_i"
  Demux10/2 -> Scope9/4  "VD1_u"
  Diode3/1 -> Demux10/1
  Demux9/2 -> Scope9/8  "VD2_u"
  PWM_Up/1 -> Mosfet2/1
  Mosfet2/1 -> Demux4/1
  Demux4/2 -> Scope9/6  "VT2_u"
  Mosfet3/1 -> Demux11/1
  Diode2/1 -> Demux9/1
  I_L1/1 -> [I_L1]  "I_L1"
  Mean1/1 -> Display39/1
  Mean/1 -> Display41/1
  Mean2/1 -> Display40/1
  Mean3/1 -> Display42/1
  Voltage Measurement2/1 -> [U_out]  "U_out"
  [U_out] -> Scope/1  "U_out"
  [I_L1] -> IL/1, Scope/2  "I_L1"
  connections:
  Uin+/RConn1 -- Mosfet3/LConn1
  Diode2/RConn1 -- C3/LConn1 -- Voltage Measurement2/LConn1 -- Uout+/RConn1 -- C1/LConn1
  Mosfet2/LConn1 -- I_L1/RConn1 -- Diode2/LConn1
  Mosfet3/RConn1 -- Diode3/RConn1 -- L1/LConn1
  Uout-/RConn1 -- C4/RConn1 -- C2/RConn1 -- Uin-/RConn1 -- Diode3/LConn1 -- Mosfet2/RConn1 -- Voltage Measurement2/LConn2
  I_L1/LConn1 -- L1/RConn1
  C3/RConn1 -- C2/LConn1 -- C1/RConn1 -- C4/LConn1
